simulink model "populationDynamics"  (R2022b)
settings: Solver=FixedStepDiscrete  StartTime=0.0  StopTime=100  RelTol=1e-3  EnableMultiTasking=on
PreLoadFcn:
  | % Parameters
  | P0 = 1e5;   % Initial Population
  | L = 1e6;    % Carrying Capacity
  | r = 1.5e-6; % Reproduction Rate
settings Model: Creator=nicholas  LastModifiedBy=bensweet
settings SolverCC: AlgebraicLoopSolver=TrustRegion
settings DataIOCC: SaveFormat=Array  SaveTime=off  ReturnWorkspaceOutputs=off  SignalLoggingName=logsOut
settings OptimizationCC: BlockReduction=off  BooleanDataType=off  ExpressionDepthLimit=2147483647  InitFltsAndDblsToZero=on  LifeSpan=inf
settings DebuggingCC: CheckExecutionContextPreStartOutputMsg=on  UnconnectedInputMsg=warning  UnconnectedOutputMsg=warning  UnconnectedLineMsg=warning  PregeneratedLibrarySubsystemCodeDiagnostic=none  SFMachineParentedDataDiag=warning
settings HardwareCC: ProdBitPerPointer=32  ProdBitPerSizeT=32  ProdBitPerPtrDiffT=32  ProdLargestAtomicFloat=None  ProdIntDivRoundTo=Undefined  ProdEndianess=Unspecified  ProdWordSize=32  ProdHWDeviceType=32-bit Generic  TargetUnknown=on
settings ModelReferenceCC: EnableRefExpFcnMdlSchedulingChecks=on  PropagateSignalLabelsOutOfModel=off
settings SFSimCC: SimUseLocalCustomCode=off
settings RTWCC: RTWUseLocalCustomCode=off  DLArmComputeVersion=19.05
settings CodeAppCC: StateflowObjectComments=on
settings GRTTargetCC: TargetFcnLib=ansi_tfl_tmw.mat  TargetLangStandard=C89/C90 (ANSI)  CombineOutputUpdateFcns=off  GRTInterface=on
settings ConfigComp: CovMetricSettings=dw  CovSaveCumulativeToWorkspaceVar=on  CovSaveSingleToWorkspaceVar=on  CovExternalEMLEnable=off  CovSFcnEnable=off

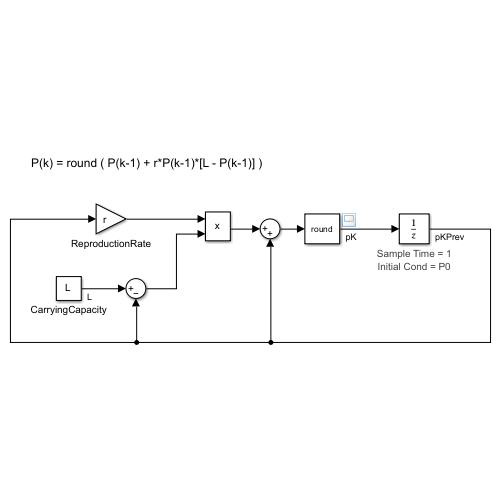
[thumbnail: Simulink's stored preview of the top-level diagram]
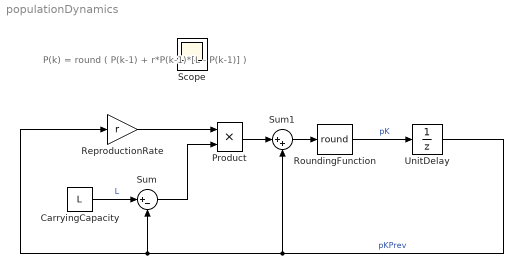
== system populationDynamics ==
  note: P(k) = round ( P(k-1) + r*P(k-1)*[L - P(k-1)] )
  CarryingCapacity : Constant  Value=L
  Product : Product  RndMeth=Zero
  ReproductionRate : Gain  Gain=r
  RoundingFunction : Rounding  Operator=round
  Sum : Sum  Inputs=|+-
  Sum1 : Sum  Inputs=|++
  UnitDelay : UnitDelay  InitialCondition=P0  HasFrameUpgradeWarning=on
      settings: AttributesFormatString=Sample Time = %<SampleTime>\nInitial Cond = %<X0>
  Scope : Scope
  wires:
  Sum/1 -> Product/2
  UnitDelay/1 -> ReproductionRate/1, Sum/2, Sum1/2  "pKPrev"
  CarryingCapacity/1 -> Sum/1  "L"
  Product/1 -> Sum1/1
  ReproductionRate/1 -> Product/1
  RoundingFunction/1 -> UnitDelay/1  "pK"
  Sum1/1 -> RoundingFunction/1
